simulink model "Bloc_regul_4position_25kHz_discret"  (R2019a)
settings: Solver=VariableStepAuto  StartTime=0.0  StopTime=Tend  RelTol=1e-3
undefined symbols (not defined in the file or in its folder): a1_f, a2_f, b0_f, b1_f, b2_f, d, d_0, d_max, d_min, d_n, Fmax, g, G_f, Jt12, Jt14, Kd_d, Kd_d_sans_int, Kddot_d, Kddot_d_sans_int, Kpi, Kr_d, Kt, Kw_d, Kw_d_sans_int, l, L_n, m, mt, pert, R, tau_ii, tau_md, tau_mi, Udc
libraries: cstblocks x8, simulink x8
settings Model: Creator=Mattia  LastModifiedBy=franc
settings DataIOCC: ReturnWorkspaceOutputs=off
settings DebuggingCC: ArithmeticOperatorsInVariantConditions=warning
settings SFSimCC: SimUseLocalCustomCode=off
settings RTWCC: RTWUseLocalCustomCode=off
settings CodeAppCC: StateflowObjectComments=on

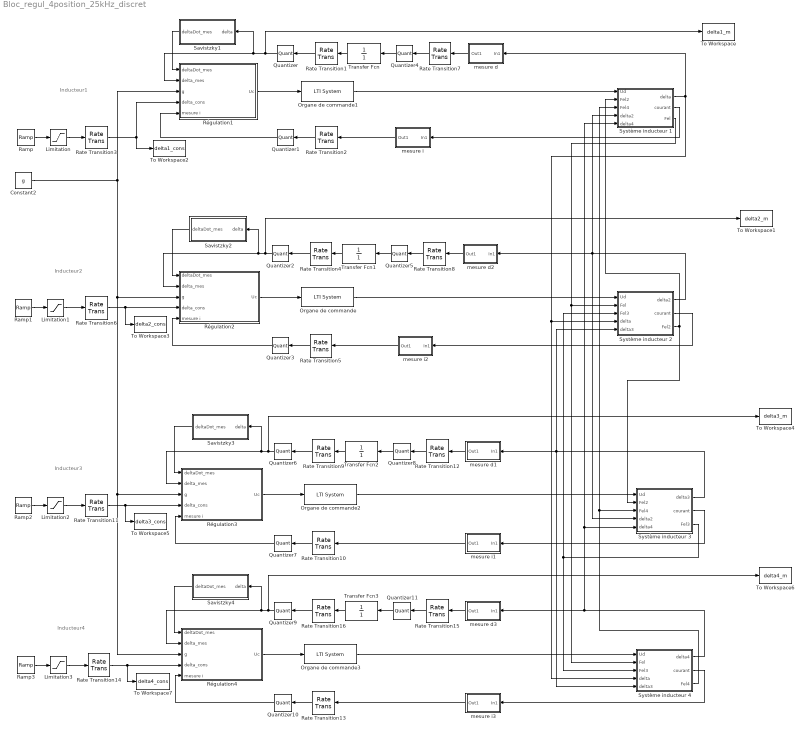
== system Bloc_regul_4position_25kHz_discret ==
  note: Inducteur2
  note: Inducteur1
  note: Inducteur3
  note: Inducteur4
  Constant2 : Constant  Value=g
  Limitation{,1..3} (4 alike) : Saturate  UpperLimit=d_0  LowerLimit=d_n
  Organe de commande{,1..3} (4 alike) : cstblocks/LTI System  sys=Gcm  IC=[]
  Quantizer{,2,6,9} (4 alike) : Quantizer  QuantizationInterval=732e-9
  Quantizer{1,3,7,10} (4 alike) : Quantizer  QuantizationInterval=0.014648438
  Quantizer{4..5,8,11} (4 alike) : Quantizer  QuantizationInterval=6.24e-6
  Ramp : simulink/Sources/Ramp  slope=-0.025  start=0  InitialOutput=d_0
  Ramp1 : simulink/Sources/Ramp  slope=-0.025  start=0.0012  InitialOutput=d_0
  Ramp2 : simulink/Sources/Ramp  slope=-0.025  start=0.4012  InitialOutput=d_0
  Ramp3 : simulink/Sources/Ramp  slope=-0.025  start=0.4  InitialOutput=d_0
  Rate Transition{1..6,9..11,13..14,16} (12 alike) : RateTransition  OutPortSampleTime=h
  Rate Transition{7..8,12,15} (4 alike) : RateTransition  OutPortSampleTime=930e-6
  Régulation1 : Subsystem
  Régulation2 : Subsystem
  Régulation3 : Subsystem
  Régulation4 : Subsystem
  Savistzky1 : Subsystem
  Savistzky2 : Subsystem
  Savistzky3 : Subsystem
  Savistzky4 : Subsystem
  Système inducteur 1 : Subsystem
  Système inducteur 2 : Subsystem
  Système inducteur 3 : Subsystem
  Système inducteur 4 : Subsystem
  To Workspace : ToWorkspace  VariableName=delta1_m  SaveFormat=Timeseries  SampleTime=-1
  To Workspace1 : ToWorkspace  VariableName=delta2_m  SaveFormat=Timeseries  SampleTime=-1
  To Workspace2 : ToWorkspace  VariableName=delta1_cons  SaveFormat=Timeseries  SampleTime=-1
  To Workspace3 : ToWorkspace  VariableName=delta2_cons  SaveFormat=Timeseries  SampleTime=-1
  To Workspace4 : ToWorkspace  VariableName=delta3_m  SaveFormat=Timeseries  SampleTime=-1
  To Workspace5 : ToWorkspace  VariableName=delta3_cons  SaveFormat=Timeseries  SampleTime=-1
  To Workspace6 : ToWorkspace  VariableName=delta4_m  SaveFormat=Timeseries  SampleTime=-1
  To Workspace7 : ToWorkspace  VariableName=delta4_cons  SaveFormat=Timeseries  SampleTime=-1
  Transfer Fcn{,1..3} (4 alike) : TransferFcn  Denominator=[1]
  "mesure d " : Subsystem
  mesure d1 : Subsystem
  mesure d2 : Subsystem
  mesure d3 : Subsystem
  mesure i : Subsystem
  mesure i1 : Subsystem
  mesure i2 : Subsystem
  mesure i3 : Subsystem
  wires:
  Ramp/1 -> Limitation/1
  Limitation/1 -> Rate Transition3/1
  Rate Transition1/1 -> Quantizer/1
  Rate Transition2/1 -> Quantizer1/1
  Limitation1/1 -> Rate Transition6/1
  Rate Transition5/1 -> Quantizer3/1
  Rate Transition4/1 -> Quantizer2/1
  Ramp1/1 -> Limitation1/1
  Quantizer3/1 -> Régulation2/5(mesure i)
  Rate Transition6/1 -> To Workspace3/1, Régulation2/4(delta_cons)
  Constant2/1 -> Régulation3/3(g), Régulation4/3(g), Régulation2/3(g), Régulation1/3(g)
  Rate Transition3/1 -> To Workspace2/1, Régulation1/4(delta_cons)
  Quantizer1/1 -> Régulation1/5(mesure i)
  mesure i/1(Out1) -> Rate Transition2/1
  mesure i2/1(Out1) -> Rate Transition5/1
  Quantizer2/1 -> To Workspace1/1, Régulation2/2(delta_mes), Savistzky2/1(delta)
  Savistzky2/1(deltaDot_mes) -> Régulation2/1(deltaDot_mes)
  Savistzky1/1(deltaDot_mes) -> Régulation1/1(deltaDot_mes)
  Système inducteur 2/2(courant) -> mesure i2/1(In1)
  Système inducteur 1/1(delta) -> Système inducteur 4/4(delta), Système inducteur 2/4(delta), "mesure d "/1(In1)
  Système inducteur 1/2(courant) -> mesure i/1(In1)
  Système inducteur 2/1(delta2) -> Système inducteur 3/4(delta2), Système inducteur 1/4(delta2), mesure d2/1(In1)
  Système inducteur 2/3(Fel2) -> Système inducteur 3/2(Fel2), Système inducteur 1/2(Fel2)
  Organe de commande/1 -> Système inducteur 2/1(Ud)
  Régulation2/1(Uc) -> Organe de commande/1
  Organe de commande1/1 -> Système inducteur 1/1(Ud)
  Régulation1/1(Uc) -> Organe de commande1/1
  Quantizer/1 -> To Workspace/1, Régulation1/2(delta_mes), Savistzky1/1(delta)
  Transfer Fcn/1 -> Rate Transition1/1
  Quantizer4/1 -> Transfer Fcn/1
  Rate Transition7/1 -> Quantizer4/1
  "mesure d "/1(Out1) -> Rate Transition7/1
  mesure d2/1(Out1) -> Rate Transition8/1
  Rate Transition8/1 -> Quantizer5/1
  Quantizer5/1 -> Transfer Fcn1/1
  Transfer Fcn1/1 -> Rate Transition4/1
  Régulation3/1(Uc) -> Organe de commande2/1
  Transfer Fcn2/1 -> Rate Transition9/1
  Rate Transition12/1 -> Quantizer8/1
  Limitation2/1 -> Rate Transition11/1
  Rate Transition10/1 -> Quantizer7/1
  mesure d1/1(Out1) -> Rate Transition12/1
  Quantizer8/1 -> Transfer Fcn2/1
  Organe de commande2/1 -> Système inducteur 3/1(Ud)
  Rate Transition9/1 -> Quantizer6/1
  Système inducteur 3/2(courant) -> mesure i1/1(In1)
  mesure i1/1(Out1) -> Rate Transition10/1
  Quantizer6/1 -> To Workspace4/1, Régulation3/2(delta_mes), Savistzky3/1(delta)
  Ramp2/1 -> Limitation2/1
  Rate Transition11/1 -> To Workspace5/1, Régulation3/4(delta_cons)
  Savistzky3/1(deltaDot_mes) -> Régulation3/1(deltaDot_mes)
  Quantizer7/1 -> Régulation3/5(mesure i)
  Quantizer10/1 -> Régulation4/5(mesure i)
  Rate Transition14/1 -> To Workspace7/1, Régulation4/4(delta_cons)
  Savistzky4/1(deltaDot_mes) -> Régulation4/1(deltaDot_mes)
  Ramp3/1 -> Limitation3/1
  Quantizer9/1 -> To Workspace6/1, Régulation4/2(delta_mes), Savistzky4/1(delta)
  mesure i3/1(Out1) -> Rate Transition13/1
  Système inducteur 4/2(courant) -> mesure i3/1(In1)
  Rate Transition16/1 -> Quantizer9/1
  Rate Transition13/1 -> Quantizer10/1
  Rate Transition15/1 -> Quantizer11/1
  Limitation3/1 -> Rate Transition14/1
  Quantizer11/1 -> Transfer Fcn3/1
  mesure d3/1(Out1) -> Rate Transition15/1
  Transfer Fcn3/1 -> Rate Transition16/1
  Organe de commande3/1 -> Système inducteur 4/1(Ud)
  Régulation4/1(Uc) -> Organe de commande3/1
  Système inducteur 4/3(Fel4) -> Système inducteur 3/3(Fel4), Système inducteur 1/3(Fel4)
  Système inducteur 4/1(delta4) -> Système inducteur 3/5(delta4), Système inducteur 1/5(delta4), mesure d3/1(In1)
  Système inducteur 1/3(Fel) -> Système inducteur 2/2(Fel), Système inducteur 4/2(Fel)
  Système inducteur 3/3(Fel3) -> Système inducteur 2/3(Fel3), Système inducteur 4/3(Fel3)
  Système inducteur 3/1(delta3) -> Système inducteur 4/5(delta3), Système inducteur 2/5(delta3), mesure d1/1(In1)

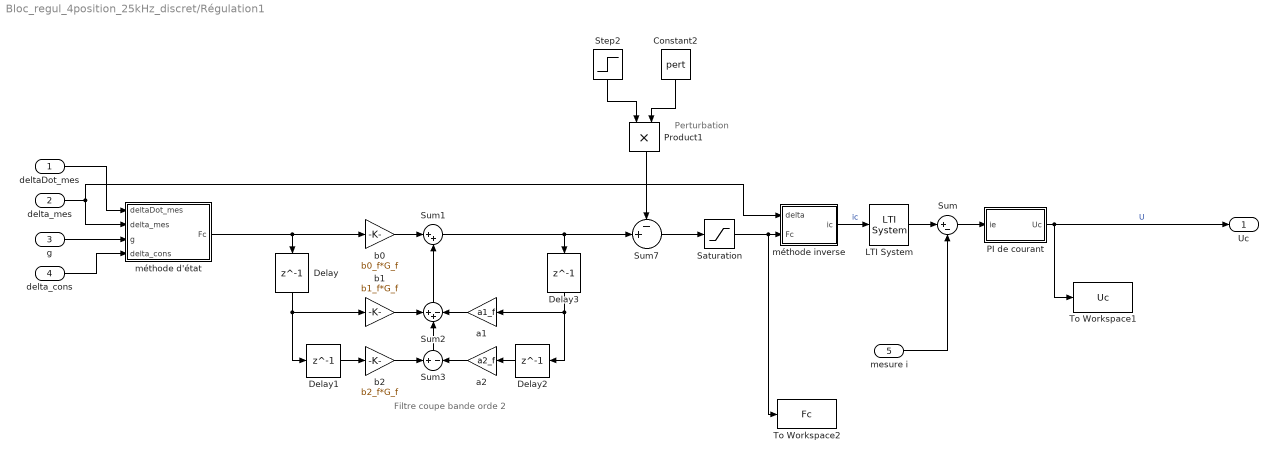
== system Bloc_regul_4position_25kHz_discret/Régulation1 ==
  note: Filtre coupe bande orde 2
  note: Perturbation
  deltaDot_mes : Inport
  delta_mes : Inport  Port=2
  g : Inport  Port=3
  delta_cons : Inport  Port=4
  mesure i : Inport  Port=5
  Constant2 : Constant  Value=pert
  Delay{,1..3} (4 alike) : Delay  DelayLength=1
  LTI System : cstblocks/LTI System  sys=tf(1,1)  IC=[]
  PI de courant : Subsystem
  Product1 : Product
  Saturation : Saturate  UpperLimit=Fmax  LowerLimit=0
  Step2 : Step  After=30  SampleTime=0
  Sum : Sum  Inputs=|+-
  Sum1 : Sum  Inputs=|++
  Sum2 : Sum  Inputs=++-
  Sum3 : Sum  Inputs=+|-
  Sum7 : Sum  Inputs=-+|
  To Workspace1 : ToWorkspace  VariableName=Uc  SaveFormat=Timeseries  SampleTime=-1
  To Workspace2 : ToWorkspace  VariableName=Fc  SaveFormat=Timeseries  SampleTime=-1
  a1 : Gain  Gain=a1_f
  a2 : Gain  Gain=a2_f
  b0 : Gain  Gain=b0_f*G_f
  b1 : Gain  Gain=b1_f*G_f
  b2 : Gain  Gain=b2_f*G_f
  méthode d'état : Subsystem
  méthode inverse : Subsystem
  Uc : Outport
  wires:
  LTI System/1 -> Sum/1
  PI de courant/1(Uc) -> Uc/1, To Workspace1/1  "U"
  Sum/1 -> PI de courant/1(ie)
  méthode inverse/1(ic) -> LTI System/1  "ic"
  mesure i/1 -> Sum/2
  g/1 -> méthode d'état/3("g ")
  delta_cons/1 -> méthode d'état/4(delta_cons)
  delta_mes/1 -> méthode d'état/2(delta_mes), méthode inverse/1(delta)
  deltaDot_mes/1 -> méthode d'état/1(deltaDot_mes)
  méthode d'état/1(Fc) -> b0/1, Delay/1
  b0/1 -> Sum1/1
  a2/1 -> Sum3/2
  Delay3/1 -> a1/1, Delay2/1
  Delay2/1 -> a2/1
  b1/1 -> Sum2/1
  a1/1 -> Sum2/3
  Sum3/1 -> Sum2/2
  Sum2/1 -> Sum1/2
  b2/1 -> Sum3/1
  Delay/1 -> b1/1, Delay1/1
  Delay1/1 -> b2/1
  Saturation/1 -> To Workspace2/1, méthode inverse/2(Fc)
  Sum7/1 -> Saturation/1
  Sum1/1 -> Sum7/2, Delay3/1
  Constant2/1 -> Product1/2
  Step2/1 -> Product1/1
  Product1/1 -> Sum7/1

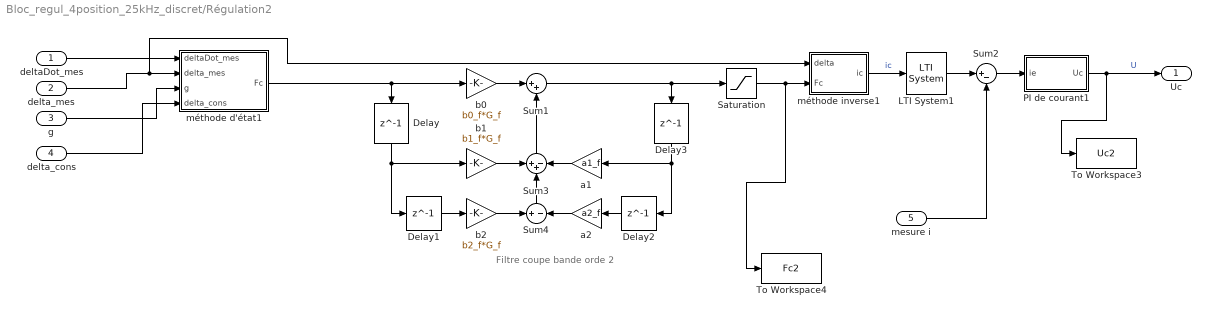
== system Bloc_regul_4position_25kHz_discret/Régulation2 ==
  note: Filtre coupe bande orde 2
  deltaDot_mes : Inport
  delta_mes : Inport  Port=2
  g : Inport  Port=3
  delta_cons : Inport  Port=4
  mesure i : Inport  Port=5
  Delay{,1..3} (4 alike) : Delay  DelayLength=1
  LTI System1 : cstblocks/LTI System  sys=tf(1,1)  IC=[]
  PI de courant1 : Subsystem
  Saturation : Saturate  UpperLimit=Fmax  LowerLimit=0
  Sum1 : Sum  Inputs=|++
  Sum2 : Sum  Inputs=|+-
  Sum3 : Sum  Inputs=++-
  Sum4 : Sum  Inputs=+|-
  To Workspace3 : ToWorkspace  VariableName=Uc2  SaveFormat=Timeseries  SampleTime=-1
  To Workspace4 : ToWorkspace  VariableName=Fc2  SaveFormat=Timeseries  SampleTime=-1
  a1 : Gain  Gain=a1_f
  a2 : Gain  Gain=a2_f
  b0 : Gain  Gain=b0_f*G_f
  b1 : Gain  Gain=b1_f*G_f
  b2 : Gain  Gain=b2_f*G_f
  méthode d'état1 : Subsystem
  méthode inverse1 : Subsystem
  Uc : Outport
  wires:
  PI de courant1/1(Uc) -> Uc/1, To Workspace3/1  "U"
  méthode inverse1/1(ic) -> LTI System1/1  "ic"
  LTI System1/1 -> Sum2/1
  Sum2/1 -> PI de courant1/1(ie)
  deltaDot_mes/1 -> méthode d'état1/1(deltaDot_mes)
  delta_mes/1 -> méthode inverse1/1(delta), méthode d'état1/2(delta_mes)
  g/1 -> méthode d'état1/3("g ")
  delta_cons/1 -> méthode d'état1/4(delta_cons)
  mesure i/1 -> Sum2/2
  b1/1 -> Sum3/1
  Sum3/1 -> Sum1/2
  Delay/1 -> b1/1, Delay1/1
  b2/1 -> Sum4/1
  a2/1 -> Sum4/2
  b0/1 -> Sum1/1
  Delay3/1 -> a1/1, Delay2/1
  Sum4/1 -> Sum3/2
  méthode d'état1/1(Fc) -> b0/1, Delay/1
  a1/1 -> Sum3/3
  Sum1/1 -> Saturation/1, Delay3/1
  Delay2/1 -> a2/1
  Delay1/1 -> b2/1
  Saturation/1 -> To Workspace4/1, méthode inverse1/2(Fc)

== system Bloc_regul_4position_25kHz_discret/Régulation3 ==
  note: Filtre coupe bande orde 2
  deltaDot_mes : Inport
  delta_mes : Inport  Port=2
  g : Inport  Port=3
  delta_cons : Inport  Port=4
  mesure i : Inport  Port=5
  Delay{,1..3} (4 alike) : Delay  DelayLength=1
  LTI System1 : cstblocks/LTI System  sys=tf(1,1)  IC=[]
  PI de courant1 : Subsystem
  Saturation : Saturate  UpperLimit=Fmax  LowerLimit=0
  Sum1 : Sum  Inputs=|++
  Sum2 : Sum  Inputs=|+-
  Sum3 : Sum  Inputs=++-
  Sum4 : Sum  Inputs=+|-
  To Workspace3 : ToWorkspace  VariableName=Uc3  SaveFormat=Timeseries  SampleTime=-1
  To Workspace4 : ToWorkspace  VariableName=Fc3  SaveFormat=Timeseries  SampleTime=-1
  a1 : Gain  Gain=a1_f
  a2 : Gain  Gain=a2_f
  b0 : Gain  Gain=b0_f*G_f
  b1 : Gain  Gain=b1_f*G_f
  b2 : Gain  Gain=b2_f*G_f
  méthode d'état1 : Subsystem
  méthode inverse1 : Subsystem
  Uc : Outport
  wires:
  PI de courant1/1(Uc) -> Uc/1, To Workspace3/1  "U"
  méthode inverse1/1(ic) -> LTI System1/1  "ic"
  LTI System1/1 -> Sum2/1
  Sum2/1 -> PI de courant1/1(ie)
  deltaDot_mes/1 -> méthode d'état1/1(deltaDot_mes)
  delta_mes/1 -> méthode inverse1/1(delta), méthode d'état1/2(delta_mes)
  g/1 -> méthode d'état1/3("g ")
  delta_cons/1 -> méthode d'état1/4(delta_cons)
  mesure i/1 -> Sum2/2
  b1/1 -> Sum3/1
  Sum3/1 -> Sum1/2
  Delay/1 -> b1/1, Delay1/1
  b2/1 -> Sum4/1
  a2/1 -> Sum4/2
  b0/1 -> Sum1/1
  Delay3/1 -> a1/1, Delay2/1
  Sum4/1 -> Sum3/2
  méthode d'état1/1(Fc) -> b0/1, Delay/1
  a1/1 -> Sum3/3
  Sum1/1 -> Saturation/1, Delay3/1
  Delay2/1 -> a2/1
  Delay1/1 -> b2/1
  Saturation/1 -> To Workspace4/1, méthode inverse1/2(Fc)

== system Bloc_regul_4position_25kHz_discret/Régulation4 ==
  note: Filtre coupe bande orde 2
  deltaDot_mes : Inport
  delta_mes : Inport  Port=2
  g : Inport  Port=3
  delta_cons : Inport  Port=4
  mesure i : Inport  Port=5
  Delay{,1..3} (4 alike) : Delay  DelayLength=1
  LTI System1 : cstblocks/LTI System  sys=tf(1,1)  IC=[]
  PI de courant1 : Subsystem
  Saturation : Saturate  UpperLimit=Fmax  LowerLimit=0
  Sum1 : Sum  Inputs=|++
  Sum2 : Sum  Inputs=|+-
  Sum3 : Sum  Inputs=++-
  Sum4 : Sum  Inputs=+|-
  To Workspace3 : ToWorkspace  VariableName=Uc4  SaveFormat=Timeseries  SampleTime=-1
  To Workspace4 : ToWorkspace  VariableName=Fc4  SaveFormat=Timeseries  SampleTime=-1
  a1 : Gain  Gain=a1_f
  a2 : Gain  Gain=a2_f
  b0 : Gain  Gain=b0_f*G_f
  b1 : Gain  Gain=b1_f*G_f
  b2 : Gain  Gain=b2_f*G_f
  méthode d'état1 : Subsystem
  méthode inverse1 : Subsystem
  Uc : Outport
  wires:
  PI de courant1/1(Uc) -> Uc/1, To Workspace3/1  "U"
  méthode inverse1/1(ic) -> LTI System1/1  "ic"
  LTI System1/1 -> Sum2/1
  Sum2/1 -> PI de courant1/1(ie)
  deltaDot_mes/1 -> méthode d'état1/1(deltaDot_mes)
  delta_mes/1 -> méthode inverse1/1(delta), méthode d'état1/2(delta_mes)
  g/1 -> méthode d'état1/3("g ")
  delta_cons/1 -> méthode d'état1/4(delta_cons)
  mesure i/1 -> Sum2/2
  b1/1 -> Sum3/1
  Sum3/1 -> Sum1/2
  Delay/1 -> b1/1, Delay1/1
  b2/1 -> Sum4/1
  a2/1 -> Sum4/2
  b0/1 -> Sum1/1
  Delay3/1 -> a1/1, Delay2/1
  Sum4/1 -> Sum3/2
  méthode d'état1/1(Fc) -> b0/1, Delay/1
  a1/1 -> Sum3/3
  Sum1/1 -> Saturation/1, Delay3/1
  Delay2/1 -> a2/1
  Delay1/1 -> b2/1
  Saturation/1 -> To Workspace4/1, méthode inverse1/2(Fc)

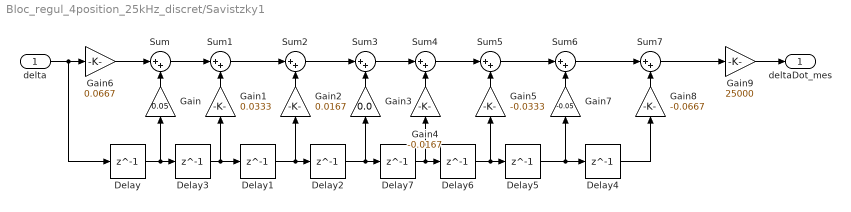
== system Bloc_regul_4position_25kHz_discret/Savistzky1 ==
  delta : Inport
  Delay{,1..7} (8 alike) : Delay  DelayLength=1
  Gain : Gain  Gain=0.05
  Gain1 : Gain  Gain=0.0333
  Gain2 : Gain  Gain=0.0167
  Gain3 : Gain  Gain=0.0
  Gain4 : Gain  Gain=-0.0167
  Gain5 : Gain  Gain=-0.0333
  Gain6 : Gain  Gain=0.0667
  Gain7 : Gain  Gain=-0.05
  Gain8 : Gain  Gain=-0.0667
  Gain9 : Gain  Gain=25000
  Sum{,1..7} (8 alike) : Sum  Inputs=|++
  deltaDot_mes : Outport
  wires:
  Delay6/1 -> Gain5/1, Delay5/1
  Delay2/1 -> Gain3/1, Delay7/1
  Gain9/1 -> deltaDot_mes/1
  Gain/1 -> Sum/2
  Sum/1 -> Sum1/1
  Gain1/1 -> Sum1/2
  Sum1/1 -> Sum2/1
  Gain2/1 -> Sum2/2
  Gain3/1 -> Sum3/2
  Sum3/1 -> Sum4/1
  Gain4/1 -> Sum4/2
  Gain5/1 -> Sum5/2
  Gain7/1 -> Sum6/2
  Gain8/1 -> Sum7/2
  Sum7/1 -> Gain9/1
  Sum6/1 -> Sum7/1
  Sum5/1 -> Sum6/1
  Sum4/1 -> Sum5/1
  Sum2/1 -> Sum3/1
  Delay/1 -> Gain/1, Delay3/1
  Delay3/1 -> Gain1/1, Delay1/1
  Delay4/1 -> Gain8/1
  Delay5/1 -> Gain7/1, Delay4/1
  Delay7/1 -> Gain4/1, Delay6/1
  Delay1/1 -> Gain2/1, Delay2/1
  delta/1 -> Gain6/1, Delay/1
  Gain6/1 -> Sum/1

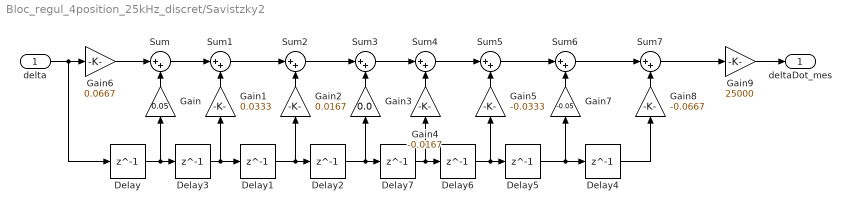
== system Bloc_regul_4position_25kHz_discret/Savistzky2 ==
  delta : Inport
  Delay{,1..7} (8 alike) : Delay  DelayLength=1
  Gain : Gain  Gain=0.05
  Gain1 : Gain  Gain=0.0333
  Gain2 : Gain  Gain=0.0167
  Gain3 : Gain  Gain=0.0
  Gain4 : Gain  Gain=-0.0167
  Gain5 : Gain  Gain=-0.0333
  Gain6 : Gain  Gain=0.0667
  Gain7 : Gain  Gain=-0.05
  Gain8 : Gain  Gain=-0.0667
  Gain9 : Gain  Gain=25000
  Sum{,1..7} (8 alike) : Sum  Inputs=|++
  deltaDot_mes : Outport
  wires:
  Delay6/1 -> Gain5/1, Delay5/1
  Delay2/1 -> Gain3/1, Delay7/1
  Gain9/1 -> deltaDot_mes/1
  Gain/1 -> Sum/2
  Sum/1 -> Sum1/1
  Gain1/1 -> Sum1/2
  Sum1/1 -> Sum2/1
  Gain2/1 -> Sum2/2
  Gain3/1 -> Sum3/2
  Sum3/1 -> Sum4/1
  Gain4/1 -> Sum4/2
  Gain5/1 -> Sum5/2
  Gain7/1 -> Sum6/2
  Gain8/1 -> Sum7/2
  Sum7/1 -> Gain9/1
  Sum6/1 -> Sum7/1
  Sum5/1 -> Sum6/1
  Sum4/1 -> Sum5/1
  Sum2/1 -> Sum3/1
  Delay/1 -> Gain/1, Delay3/1
  Delay3/1 -> Gain1/1, Delay1/1
  Delay4/1 -> Gain8/1
  Delay5/1 -> Gain7/1, Delay4/1
  Delay7/1 -> Gain4/1, Delay6/1
  Delay1/1 -> Gain2/1, Delay2/1
  delta/1 -> Gain6/1, Delay/1
  Gain6/1 -> Sum/1

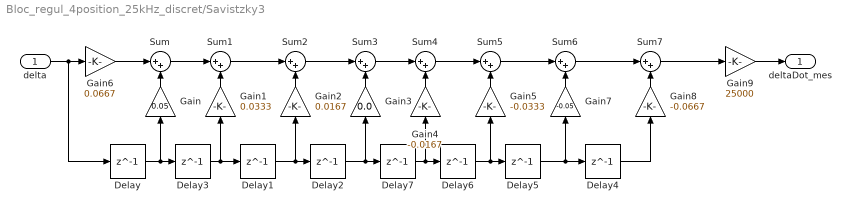
== system Bloc_regul_4position_25kHz_discret/Savistzky3 ==
  delta : Inport
  Delay{,1..7} (8 alike) : Delay  DelayLength=1
  Gain : Gain  Gain=0.05
  Gain1 : Gain  Gain=0.0333
  Gain2 : Gain  Gain=0.0167
  Gain3 : Gain  Gain=0.0
  Gain4 : Gain  Gain=-0.0167
  Gain5 : Gain  Gain=-0.0333
  Gain6 : Gain  Gain=0.0667
  Gain7 : Gain  Gain=-0.05
  Gain8 : Gain  Gain=-0.0667
  Gain9 : Gain  Gain=25000
  Sum{,1..7} (8 alike) : Sum  Inputs=|++
  deltaDot_mes : Outport
  wires:
  Delay6/1 -> Gain5/1, Delay5/1
  Delay2/1 -> Gain3/1, Delay7/1
  Gain9/1 -> deltaDot_mes/1
  Gain/1 -> Sum/2
  Sum/1 -> Sum1/1
  Gain1/1 -> Sum1/2
  Sum1/1 -> Sum2/1
  Gain2/1 -> Sum2/2
  Gain3/1 -> Sum3/2
  Sum3/1 -> Sum4/1
  Gain4/1 -> Sum4/2
  Gain5/1 -> Sum5/2
  Gain7/1 -> Sum6/2
  Gain8/1 -> Sum7/2
  Sum7/1 -> Gain9/1
  Sum6/1 -> Sum7/1
  Sum5/1 -> Sum6/1
  Sum4/1 -> Sum5/1
  Sum2/1 -> Sum3/1
  Delay/1 -> Gain/1, Delay3/1
  Delay3/1 -> Gain1/1, Delay1/1
  Delay4/1 -> Gain8/1
  Delay5/1 -> Gain7/1, Delay4/1
  Delay7/1 -> Gain4/1, Delay6/1
  Delay1/1 -> Gain2/1, Delay2/1
  delta/1 -> Gain6/1, Delay/1
  Gain6/1 -> Sum/1

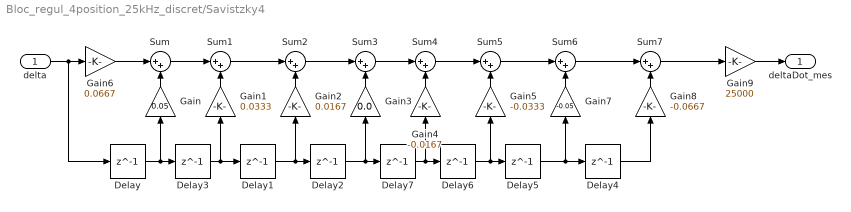
== system Bloc_regul_4position_25kHz_discret/Savistzky4 ==
  delta : Inport
  Delay{,1..7} (8 alike) : Delay  DelayLength=1
  Gain : Gain  Gain=0.05
  Gain1 : Gain  Gain=0.0333
  Gain2 : Gain  Gain=0.0167
  Gain3 : Gain  Gain=0.0
  Gain4 : Gain  Gain=-0.0167
  Gain5 : Gain  Gain=-0.0333
  Gain6 : Gain  Gain=0.0667
  Gain7 : Gain  Gain=-0.05
  Gain8 : Gain  Gain=-0.0667
  Gain9 : Gain  Gain=25000
  Sum{,1..7} (8 alike) : Sum  Inputs=|++
  deltaDot_mes : Outport
  wires:
  Delay6/1 -> Gain5/1, Delay5/1
  Delay2/1 -> Gain3/1, Delay7/1
  Gain9/1 -> deltaDot_mes/1
  Gain/1 -> Sum/2
  Sum/1 -> Sum1/1
  Gain1/1 -> Sum1/2
  Sum1/1 -> Sum2/1
  Gain2/1 -> Sum2/2
  Gain3/1 -> Sum3/2
  Sum3/1 -> Sum4/1
  Gain4/1 -> Sum4/2
  Gain5/1 -> Sum5/2
  Gain7/1 -> Sum6/2
  Gain8/1 -> Sum7/2
  Sum7/1 -> Gain9/1
  Sum6/1 -> Sum7/1
  Sum5/1 -> Sum6/1
  Sum4/1 -> Sum5/1
  Sum2/1 -> Sum3/1
  Delay/1 -> Gain/1, Delay3/1
  Delay3/1 -> Gain1/1, Delay1/1
  Delay4/1 -> Gain8/1
  Delay5/1 -> Gain7/1, Delay4/1
  Delay7/1 -> Gain4/1, Delay6/1
  Delay1/1 -> Gain2/1, Delay2/1
  delta/1 -> Gain6/1, Delay/1
  Gain6/1 -> Sum/1

== system Bloc_regul_4position_25kHz_discret/Système inducteur 1 ==
  Ud : Inport
  Fel2 : Inport  Port=2
  Fel4 : Inport  Port=3
  delta2 : Inport  Port=4
  delta4 : Inport  Port=5
  Partie Electrique : Subsystem
  Partie Mécanique : Subsystem
  delta : Outport
  courant : Outport  Port=2
  Fel : Outport  Port=3
  wires:
  Ud/1 -> Partie Electrique/1(Ud)
  Partie Mécanique/2(delta) -> Partie Electrique/3(delta), delta/1
  Partie Electrique/1(i) -> courant/1
  Partie Mécanique/1(deltaDot) -> Partie Electrique/2(deltaDot)
  Partie Electrique/2(Fel) -> Fel/1, Partie Mécanique/1(Fel)
  Fel2/1 -> Partie Mécanique/2(Fel2)
  delta2/1 -> Partie Mécanique/4(delta2)
  Fel4/1 -> Partie Mécanique/3(Fel4)
  delta4/1 -> Partie Mécanique/5(delta4)

== system Bloc_regul_4position_25kHz_discret/Système inducteur 2 ==
  Ud : Inport
  Fel : Inport  Port=2
  Fel3 : Inport  Port=3
  delta : Inport  Port=4
  delta3 : Inport  Port=5
  Partie Electrique : Subsystem
  Partie Mécanique2 : Subsystem
  delta2 : Outport
  courant : Outport  Port=2
  Fel2 : Outport  Port=3
  wires:
  Ud/1 -> Partie Electrique/1(Ud)
  Partie Mécanique2/2(delta2) -> Partie Electrique/3(delta), delta2/1
  Partie Electrique/1(i2) -> courant/1
  Partie Mécanique2/1(deltaDot2) -> Partie Electrique/2(deltaDot)
  Partie Electrique/2(Fel2) -> Fel2/1, Partie Mécanique2/2(Fel2)
  Fel/1 -> Partie Mécanique2/1(Fel)
  delta/1 -> Partie Mécanique2/4(Delta)
  Fel3/1 -> Partie Mécanique2/3(Fel3)
  delta3/1 -> Partie Mécanique2/5(Delta3)

== system Bloc_regul_4position_25kHz_discret/Système inducteur 3 ==
  Ud : Inport
  Fel2 : Inport  Port=2
  Fel4 : Inport  Port=3
  delta2 : Inport  Port=4
  delta4 : Inport  Port=5
  Partie Electrique : Subsystem
  Partie Mécanique2 : Subsystem
  delta3 : Outport
  courant : Outport  Port=2
  Fel3 : Outport  Port=3
  wires:
  Ud/1 -> Partie Electrique/1(Ud)
  Partie Mécanique2/2(delta3) -> Partie Electrique/3(delta), delta3/1
  Partie Electrique/1(i3) -> courant/1
  Partie Mécanique2/1(deltaDot3) -> Partie Electrique/2(deltaDot)
  Partie Electrique/2(Fel3) -> Fel3/1, Partie Mécanique2/2(Fel3)
  Fel2/1 -> Partie Mécanique2/1(Fel2)
  delta2/1 -> Partie Mécanique2/4(Delta2)
  Fel4/1 -> Partie Mécanique2/3(Fel4)
  delta4/1 -> Partie Mécanique2/5(Delta4)

== system Bloc_regul_4position_25kHz_discret/Système inducteur 4 ==
  Ud : Inport
  Fel : Inport  Port=2
  Fel3 : Inport  Port=3
  delta : Inport  Port=4
  delta3 : Inport  Port=5
  Partie Electrique : Subsystem
  Partie Mécanique2 : Subsystem
  delta4 : Outport
  courant : Outport  Port=2
  Fel4 : Outport  Port=3
  wires:
  Ud/1 -> Partie Electrique/1(Ud)
  Partie Mécanique2/2(delta4) -> Partie Electrique/3(delta), delta4/1
  Partie Electrique/1(i4) -> courant/1
  Partie Mécanique2/1(deltaDot4) -> Partie Electrique/2(deltaDot)
  Partie Electrique/2(Fel4) -> Partie Mécanique2/3(Fel4), Fel4/1
  Fel/1 -> Partie Mécanique2/1(Fel)
  delta/1 -> Partie Mécanique2/4(Delta)
  Fel3/1 -> Partie Mécanique2/2(Fel3)
  delta3/1 -> Partie Mécanique2/5(Delta3)

== system Bloc_regul_4position_25kHz_discret/mesure d  ==
  In1 : Inport
  Gain : Gain  Gain=1/tau_md
  Integrator : Integrator  InitialCondition=d_0
  Sum : Sum  Inputs=|+-
  Out1 : Outport
  wires:
  Gain/1 -> Integrator/1
  Integrator/1 -> Sum/2, Out1/1
  In1/1 -> Sum/1
  Sum/1 -> Gain/1

== system Bloc_regul_4position_25kHz_discret/mesure d1 ==
  In1 : Inport
  Gain : Gain  Gain=1/tau_md
  Integrator : Integrator  InitialCondition=d_0
  Sum : Sum  Inputs=|+-
  Out1 : Outport
  wires:
  Gain/1 -> Integrator/1
  Integrator/1 -> Sum/2, Out1/1
  In1/1 -> Sum/1
  Sum/1 -> Gain/1

== system Bloc_regul_4position_25kHz_discret/mesure d2 ==
  In1 : Inport
  Gain : Gain  Gain=1/tau_md
  Integrator : Integrator  InitialCondition=d_0
  Sum : Sum  Inputs=|+-
  Out1 : Outport
  wires:
  Gain/1 -> Integrator/1
  Integrator/1 -> Sum/2, Out1/1
  In1/1 -> Sum/1
  Sum/1 -> Gain/1

== system Bloc_regul_4position_25kHz_discret/mesure d3 ==
  In1 : Inport
  Gain : Gain  Gain=1/tau_md
  Integrator : Integrator  InitialCondition=d_0
  Sum : Sum  Inputs=|+-
  Out1 : Outport
  wires:
  Gain/1 -> Integrator/1
  Integrator/1 -> Sum/2, Out1/1
  In1/1 -> Sum/1
  Sum/1 -> Gain/1

== system Bloc_regul_4position_25kHz_discret/mesure i ==
  In1 : Inport
  Gain : Gain  Gain=1/tau_mi
  Integrator : Integrator
  Sum : Sum  Inputs=|+-
  Out1 : Outport
  wires:
  Gain/1 -> Integrator/1
  In1/1 -> Sum/1
  Integrator/1 -> Sum/2, Out1/1
  Sum/1 -> Gain/1

== system Bloc_regul_4position_25kHz_discret/mesure i1 ==
  In1 : Inport
  Gain : Gain  Gain=1/tau_mi
  Integrator : Integrator
  Sum : Sum  Inputs=|+-
  Out1 : Outport
  wires:
  Gain/1 -> Integrator/1
  In1/1 -> Sum/1
  Integrator/1 -> Sum/2, Out1/1
  Sum/1 -> Gain/1

== system Bloc_regul_4position_25kHz_discret/mesure i2 ==
  In1 : Inport
  Gain : Gain  Gain=1/tau_mi
  Integrator : Integrator
  Sum : Sum  Inputs=|+-
  Out1 : Outport
  wires:
  Gain/1 -> Integrator/1
  In1/1 -> Sum/1
  Integrator/1 -> Sum/2, Out1/1
  Sum/1 -> Gain/1

== system Bloc_regul_4position_25kHz_discret/mesure i3 ==
  In1 : Inport
  Gain : Gain  Gain=1/tau_mi
  Integrator : Integrator
  Sum : Sum  Inputs=|+-
  Out1 : Outport
  wires:
  Gain/1 -> Integrator/1
  In1/1 -> Sum/1
  Integrator/1 -> Sum/2, Out1/1
  Sum/1 -> Gain/1

== system Bloc_regul_4position_25kHz_discret/Régulation1/PI de courant ==
  ie : Inport
  Gain : Gain  Gain=Kpi
  Gain1 : Gain  Gain=1/tau_ii
  Integrator : Integrator
  Saturation : Saturate  UpperLimit=Udc  LowerLimit=0
  Sum : Sum  Inputs=|++
  Sum1 : Sum  Inputs=|+-
  Sum4 : Sum  Inputs=+|-
  Uc : Outport
  wires:
  Sum1/1 -> Gain1/1
  Saturation/1 -> Sum4/2, Uc/1
  Sum/1 -> Saturation/1, Sum4/1
  Integrator/1 -> Sum/2
  Gain/1 -> Sum1/1, Sum/1
  Gain1/1 -> Integrator/1
  Sum4/1 -> Sum1/2
  ie/1 -> Gain/1

== system Bloc_regul_4position_25kHz_discret/Régulation1/méthode d'état ==
  deltaDot_mes : Inport
  delta_mes : Inport  Port=2
  "g " : Inport  Port=3
  delta_cons : Inport  Port=4
  Delay : Delay  DelayLength=1  InitialCondition=0
  Gain : Gain  Gain=m
  Gain1 : Gain  Gain=Kw_d
  Gain2 : Gain  Gain=Kr_d
  Gain3 : Gain  Gain=Kddot_d
  Gain4 : Gain  Gain=Kd_d
  Gain5 : Gain  Gain=1/Kw_d
  Saturation : Saturate  UpperLimit=Fmax  LowerLimit=0
  Sum : Sum  Inputs=+++
  Sum1 : Sum  Inputs=+-
  Sum2 : Sum  Inputs=|++
  Sum3 : Sum  Inputs=+-|
  Sum4 : Sum  Inputs=+|-
  Sum5 : Sum  Inputs=|+-
  Sum6 : Sum  Inputs=|++
  To Workspace1 : ToWorkspace  VariableName=Reg_cons  SaveFormat=Timeseries  SampleTime=-1
  To Workspace2 : ToWorkspace  VariableName=MG  SaveFormat=Timeseries  SampleTime=-1
  To Workspace3 : ToWorkspace  VariableName=Integrateur  SaveFormat=Timeseries  SampleTime=-1
  To Workspace4 : ToWorkspace  VariableName=Fc_reg  SaveFormat=Timeseries  SampleTime=-1
  Fc : Outport
  wires:
  Sum5/1 -> Sum6/1
  deltaDot_mes/1 -> Gain3/1
  delta_mes/1 -> Gain4/1, Sum1/2
  delta_cons/1 -> Sum1/1, Gain1/1
  Delay/1 -> Sum6/2, Gain2/1
  "g "/1 -> Gain/1
  Saturation/1 -> Fc/1, Sum4/2
  Sum6/1 -> Delay/1
  Gain4/1 -> Sum2/1
  Gain2/1 -> Sum3/1
  Gain/1 -> Sum/1, To Workspace2/1
  Gain3/1 -> Sum2/2
  Gain5/1 -> Sum5/2
  Sum2/1 -> Sum3/2
  Sum4/1 -> Gain5/1
  Sum3/1 -> To Workspace3/1, Sum/3
  Sum1/1 -> Sum5/1
  Gain1/1 -> To Workspace1/1, Sum/2
  Sum/1 -> To Workspace4/1, Sum4/1, Saturation/1

== system Bloc_regul_4position_25kHz_discret/Régulation1/méthode inverse ==
  delta : Inport
  Fc : Inport  Port=2
  Gain : Gain  Gain=2/(L_n*d_n)
  Product : Product
  Sqrt : Sqrt  OutputSignalType=real  SaturateOnIntegerOverflow=on
  ic : Outport
  wires:
  Gain/1 -> Sqrt/1
  Fc/1 -> Gain/1
  delta/1 -> Product/1
  Product/1 -> ic/1
  Sqrt/1 -> Product/2

== system Bloc_regul_4position_25kHz_discret/Régulation2/PI de courant1 ==
  ie : Inport
  Gain : Gain  Gain=Kpi
  Gain1 : Gain  Gain=1/tau_ii
  Integrator : Integrator
  Saturation : Saturate  UpperLimit=Udc  LowerLimit=0
  Sum : Sum  Inputs=|++
  Sum1 : Sum  Inputs=|+-
  Sum4 : Sum  Inputs=+|-
  Uc : Outport
  wires:
  Sum1/1 -> Gain1/1
  Saturation/1 -> Sum4/2, Uc/1
  Sum/1 -> Saturation/1, Sum4/1
  Integrator/1 -> Sum/2
  Gain/1 -> Sum1/1, Sum/1
  Gain1/1 -> Integrator/1
  Sum4/1 -> Sum1/2
  ie/1 -> Gain/1

== system Bloc_regul_4position_25kHz_discret/Régulation2/méthode d'état1 ==
  deltaDot_mes : Inport
  delta_mes : Inport  Port=2
  "g " : Inport  Port=3
  delta_cons : Inport  Port=4
  Delay : Delay  DelayLength=1  InitialCondition=0
  Gain : Gain  Gain=m
  Gain1 : Gain  Gain=Kw_d
  Gain2 : Gain  Gain=Kr_d
  Gain3 : Gain  Gain=Kddot_d
  Gain4 : Gain  Gain=Kd_d
  Gain5 : Gain  Gain=1/Kw_d
  Saturation : Saturate  UpperLimit=Fmax  LowerLimit=0
  Sum : Sum  Inputs=+++
  Sum1 : Sum  Inputs=+-
  Sum2 : Sum  Inputs=|++
  Sum3 : Sum  Inputs=+-|
  Sum4 : Sum  Inputs=+|-
  Sum5 : Sum  Inputs=|+-
  Sum6 : Sum  Inputs=|++
  Fc : Outport
  wires:
  Sum5/1 -> Sum6/1
  deltaDot_mes/1 -> Gain3/1
  delta_mes/1 -> Gain4/1, Sum1/2
  delta_cons/1 -> Sum1/1, Gain1/1
  Delay/1 -> Sum6/2, Gain2/1
  "g "/1 -> Gain/1
  Saturation/1 -> Fc/1, Sum4/2
  Sum6/1 -> Delay/1
  Gain4/1 -> Sum2/1
  Gain2/1 -> Sum3/1
  Gain/1 -> Sum/1
  Gain3/1 -> Sum2/2
  Gain5/1 -> Sum5/2
  Sum2/1 -> Sum3/2
  Sum4/1 -> Gain5/1
  Sum3/1 -> Sum/3
  Sum1/1 -> Sum5/1
  Gain1/1 -> Sum/2
  Sum/1 -> Sum4/1, Saturation/1

== system Bloc_regul_4position_25kHz_discret/Régulation2/méthode inverse1 ==
  delta : Inport
  Fc : Inport  Port=2
  Gain : Gain  Gain=2/(L_n*d_n)
  Product : Product
  Sqrt : Sqrt  OutputSignalType=real  SaturateOnIntegerOverflow=on
  ic : Outport
  wires:
  Gain/1 -> Sqrt/1
  Fc/1 -> Gain/1
  delta/1 -> Product/1
  Product/1 -> ic/1
  Sqrt/1 -> Product/2

== system Bloc_regul_4position_25kHz_discret/Régulation3/PI de courant1 ==
  ie : Inport
  Gain : Gain  Gain=Kpi
  Gain1 : Gain  Gain=1/tau_ii
  Integrator : Integrator
  Saturation : Saturate  UpperLimit=Udc  LowerLimit=0
  Sum : Sum  Inputs=|++
  Sum1 : Sum  Inputs=|+-
  Sum4 : Sum  Inputs=+|-
  Uc : Outport
  wires:
  Sum1/1 -> Gain1/1
  Saturation/1 -> Sum4/2, Uc/1
  Sum/1 -> Saturation/1, Sum4/1
  Integrator/1 -> Sum/2
  Gain/1 -> Sum1/1, Sum/1
  Gain1/1 -> Integrator/1
  Sum4/1 -> Sum1/2
  ie/1 -> Gain/1

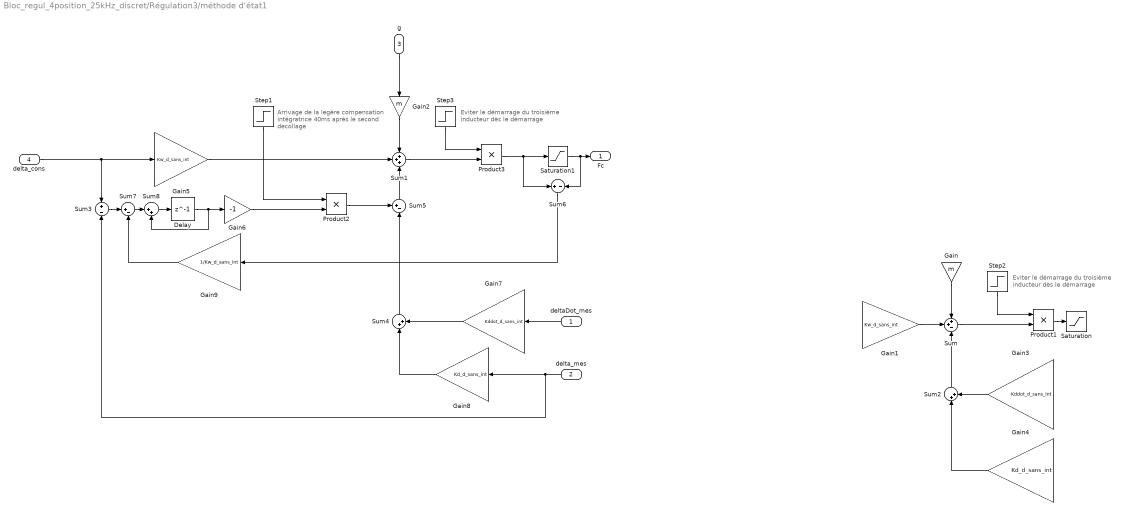
== system Bloc_regul_4position_25kHz_discret/Régulation3/méthode d'état1 ==
  note: Eviter le démarrage du troisième
      | inducteur dès le démarrage
  note: Eviter le démarrage du troisième
      | inducteur dès le démarrage
  note: Arrivage de la legère compensation
      | intégratrice 40ms après le second
      | decollage
  deltaDot_mes : Inport
  delta_mes : Inport  Port=2
  "g " : Inport  Port=3
  delta_cons : Inport  Port=4
  Delay : Delay  DelayLength=1  InitialCondition=0
  Gain : Gain  Gain=m
  Gain1 : Gain  Gain=Kw_d_sans_int
  Gain2 : Gain  Gain=m
  Gain3 : Gain  Gain=Kddot_d_sans_int
  Gain4 : Gain  Gain=Kd_d_sans_int
  Gain5 : Gain  Gain=Kw_d_sans_int
  Gain6 : Gain  Gain=-1
  Gain7 : Gain  Gain=Kddot_d_sans_int
  Gain8 : Gain  Gain=Kd_d_sans_int
  Gain9 : Gain  Gain=1/Kw_d_sans_int
  Product1 : Product
  Product2 : Product
  Product3 : Product
  Saturation : Saturate  UpperLimit=Fmax  LowerLimit=0
  Saturation1 : Saturate  UpperLimit=Fmax  LowerLimit=0
  Step1 : Step  Time=0.440  SampleTime=0
  Step2 : Step  Time=0.4  SampleTime=0
  Step3 : Step  Time=0.4  SampleTime=0
  Sum : Sum  Inputs=++-
  Sum1 : Sum  Inputs=+++
  Sum2 : Sum  Inputs=|++
  Sum3 : Sum  Inputs=+-
  Sum4 : Sum  Inputs=|++
  Sum5 : Sum  Inputs=+-|
  Sum6 : Sum  Inputs=+|-
  Sum7 : Sum  Inputs=|+-
  Sum8 : Sum  Inputs=|++
  Fc : Outport
  wires:
  "g "/1 -> Gain2/1
  deltaDot_mes/1 -> Gain7/1
  Sum8/1 -> Delay/1
  delta_mes/1 -> Sum3/2, Gain8/1
  delta_cons/1 -> Gain5/1, Sum3/1
  Sum4/1 -> Sum5/2
  Sum5/1 -> Sum1/3
  Sum7/1 -> Sum8/1
  Delay/1 -> Sum8/2, Gain6/1
  Gain2/1 -> Sum1/1
  Gain9/1 -> Sum7/2
  Gain8/1 -> Sum4/1
  Gain5/1 -> Sum1/2
  Sum3/1 -> Sum7/1
  Sum6/1 -> Gain9/1
  Gain7/1 -> Sum4/2
  Sum1/1 -> Product3/2
  Step3/1 -> Product3/1
  Product3/1 -> Sum6/1, Saturation1/1
  Product1/1 -> Saturation/1
  ? -> Gain1/1
  ? -> Gain3/1
  Gain3/1 -> Sum2/2
  Sum/1 -> Product1/2
  Sum2/1 -> Sum/3
  ? -> Gain4/1
  Gain1/1 -> Sum/2
  Gain4/1 -> Sum2/1
  Step2/1 -> Product1/1
  Gain/1 -> Sum/1
  ? -> Gain/1
  Saturation1/1 -> Sum6/2, Fc/1
  Step1/1 -> Product2/1
  Gain6/1 -> Product2/2
  Product2/1 -> Sum5/1

== system Bloc_regul_4position_25kHz_discret/Régulation3/méthode inverse1 ==
  delta : Inport
  Fc : Inport  Port=2
  Gain : Gain  Gain=2/(L_n*d_n)
  Product : Product
  Sqrt : Sqrt  OutputSignalType=real  SaturateOnIntegerOverflow=on
  ic : Outport
  wires:
  Gain/1 -> Sqrt/1
  Fc/1 -> Gain/1
  delta/1 -> Product/1
  Product/1 -> ic/1
  Sqrt/1 -> Product/2

== system Bloc_regul_4position_25kHz_discret/Régulation4/PI de courant1 ==
  ie : Inport
  Gain : Gain  Gain=Kpi
  Gain1 : Gain  Gain=1/tau_ii
  Integrator : Integrator
  Saturation : Saturate  UpperLimit=Udc  LowerLimit=0
  Sum : Sum  Inputs=|++
  Sum1 : Sum  Inputs=|+-
  Sum4 : Sum  Inputs=+|-
  Uc : Outport
  wires:
  Sum1/1 -> Gain1/1
  Saturation/1 -> Sum4/2, Uc/1
  Sum/1 -> Saturation/1, Sum4/1
  Integrator/1 -> Sum/2
  Gain/1 -> Sum1/1, Sum/1
  Gain1/1 -> Integrator/1
  Sum4/1 -> Sum1/2
  ie/1 -> Gain/1

== system Bloc_regul_4position_25kHz_discret/Régulation4/méthode d'état1 ==
  deltaDot_mes : Inport
  delta_mes : Inport  Port=2
  "g " : Inport  Port=3
  delta_cons : Inport  Port=4
  Delay : Delay  DelayLength=1  InitialCondition=0
  Gain : Gain  Gain=m
  Gain1 : Gain  Gain=Kw_d
  Gain2 : Gain  Gain=Kr_d
  Gain3 : Gain  Gain=Kddot_d
  Gain4 : Gain  Gain=Kd_d
  Gain5 : Gain  Gain=1/Kw_d
  Saturation : Saturate  UpperLimit=Fmax  LowerLimit=0
  Sum : Sum  Inputs=+++
  Sum1 : Sum  Inputs=+-
  Sum2 : Sum  Inputs=|++
  Sum3 : Sum  Inputs=+-|
  Sum4 : Sum  Inputs=+|-
  Sum5 : Sum  Inputs=|+-
  Sum6 : Sum  Inputs=|++
  Fc : Outport
  wires:
  Sum5/1 -> Sum6/1
  deltaDot_mes/1 -> Gain3/1
  delta_mes/1 -> Gain4/1, Sum1/2
  delta_cons/1 -> Sum1/1, Gain1/1
  Delay/1 -> Sum6/2, Gain2/1
  "g "/1 -> Gain/1
  Saturation/1 -> Fc/1, Sum4/2
  Sum6/1 -> Delay/1
  Gain4/1 -> Sum2/1
  Gain2/1 -> Sum3/1
  Gain/1 -> Sum/1
  Gain3/1 -> Sum2/2
  Gain5/1 -> Sum5/2
  Sum2/1 -> Sum3/2
  Sum4/1 -> Gain5/1
  Sum3/1 -> Sum/3
  Sum1/1 -> Sum5/1
  Gain1/1 -> Sum/2
  Sum/1 -> Sum4/1, Saturation/1

== system Bloc_regul_4position_25kHz_discret/Régulation4/méthode inverse1 ==
  delta : Inport
  Fc : Inport  Port=2
  Gain : Gain  Gain=2/(L_n*d_n)
  Product : Product
  Sqrt : Sqrt  OutputSignalType=real  SaturateOnIntegerOverflow=on
  ic : Outport
  wires:
  Gain/1 -> Sqrt/1
  Fc/1 -> Gain/1
  delta/1 -> Product/1
  Product/1 -> ic/1
  Sqrt/1 -> Product/2

== system Bloc_regul_4position_25kHz_discret/Système inducteur 1/Partie Electrique ==
  Ud : Inport
  deltaDot : Inport  Port=2
  delta : Inport  Port=3
  Divide : Product  Inputs=*/  CollapseMode=Specified dimension
  Gain : Gain  Gain=R
  Gain1 : Gain  Gain=1/(L_n*d_n)
  Gain3 : Gain  Gain=L_n*d_n/2
  Integrator : Integrator
  Product : Product
  Product1 : Product
  Square : Math  Operator=square  RndMeth=Zero  SaturateOnIntegerOverflow=on
  Sum : Sum  Inputs=-+|
  Sum1 : Sum  Inputs=|++
  To Workspace1 : ToWorkspace  VariableName=Fel  SaveFormat=Timeseries  SampleTime=-1
  To Workspace3 : ToWorkspace  VariableName=i  SaveFormat=Timeseries  SampleTime=-1
  i : Outport
  Fel : Outport  Port=2
  wires:
  deltaDot/1 -> Product1/2  "deltaDot"
  Gain/1 -> Sum/1
  Ud/1 -> Sum/2  "Ud"
  Divide/1 -> Square/1, Product1/1
  Product1/1 -> Sum1/2
  Gain1/1 -> Product/1
  Integrator/1 -> To Workspace3/1, i/1, Divide/1, Gain/1  "i"
  Sum1/1 -> Integrator/1  "di/dt"
  Product/1 -> Sum1/1
  Sum/1 -> Gain1/1
  Square/1 -> Gain3/1
  delta/1 -> Product/2, Divide/2  "delta"
  Gain3/1 -> To Workspace1/1, Fel/1  "Fel"

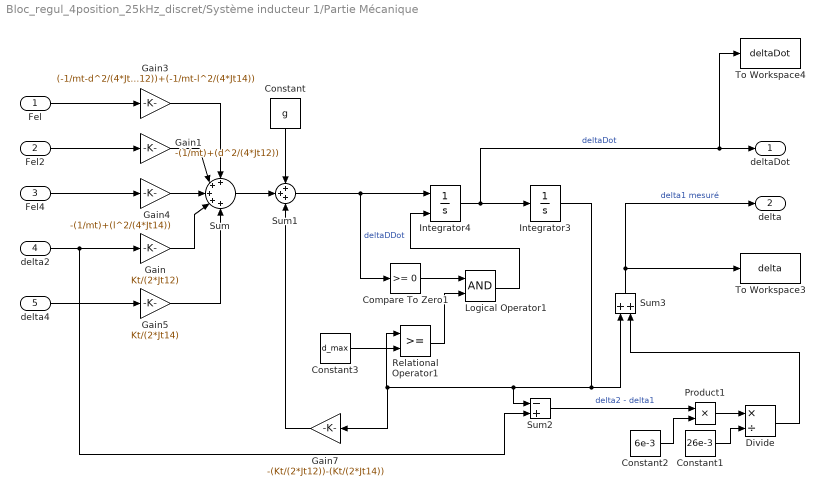
== system Bloc_regul_4position_25kHz_discret/Système inducteur 1/Partie Mécanique ==
  Fel : Inport
  Fel2 : Inport  Port=2
  Fel4 : Inport  Port=3
  delta2 : Inport  Port=4
  delta4 : Inport  Port=5
  Compare To Zero1 : simulink/Logic and Bit Operations/Compare To Zero  relop=>=  OutDataTypeStr=boolean
  Constant : Constant  Value=g
  Constant1 : Constant  Value=26e-3
  Constant2 : Constant  Value=6e-3
  Constant3 : Constant  Value=d_max
  Divide : Product  Inputs=*/
  Gain : Gain  Gain=Kt/(2*Jt12)
  Gain1 : Gain  Gain=-(1/mt)+(d^2/(4*Jt12))
  Gain3 : Gain  Gain=(-1/mt-d^2/(4*Jt12))+(-1/mt-l^2/(4*Jt14))
  Gain4 : Gain  Gain=-(1/mt)+(l^2/(4*Jt14))
  Gain5 : Gain  Gain=Kt/(2*Jt14)
  Gain7 : Gain  Gain=-(Kt/(2*Jt12))-(Kt/(2*Jt14))
  Integrator3 : Integrator  InitialCondition=d_0  LimitOutput=on  UpperSaturationLimit=d_max  LowerSaturationLimit=d_min
  Integrator4 : Integrator  ExternalReset=level  UpperSaturationLimit=0
  Logical Operator1 : Logic  AllPortsSameDT=off  OutDataTypeStr=boolean
  Product1 : Product
  Relational Operator1 : RelationalOperator  OutDataTypeStr=boolean  RndMeth=Simplest
  Sum : Sum  Inputs=+++++
  Sum1 : Sum  Inputs=+++
  Sum2 : Sum  Inputs=-+
  Sum3 : Sum
  To Workspace3 : ToWorkspace  VariableName=delta  SaveFormat=Timeseries  SampleTime=-1
  To Workspace4 : ToWorkspace  VariableName=deltaDot  SaveFormat=Timeseries  SampleTime=-1
  deltaDot : Outport
  delta : Outport  Port=2
  wires:
  Sum1/1 -> Compare To Zero1/1, Integrator4/1  "deltaDDot"
  Integrator4/1 -> To Workspace4/1, deltaDot/1, Integrator3/1  "deltaDot"
  Integrator3/1 -> Sum3/1, Sum2/1, Gain7/1, Relational Operator1/1
  Constant3/1 -> Relational Operator1/2
  Compare To Zero1/1 -> Logical Operator1/1
  Logical Operator1/1 -> Integrator4/2
  Relational Operator1/1 -> Logical Operator1/2
  Gain7/1 -> Sum1/3
  Constant/1 -> Sum1/1
  Sum/1 -> Sum1/2
  Gain1/1 -> Sum/2
  Fel2/1 -> Gain1/1
  delta2/1 -> Sum2/2, Gain/1
  Gain/1 -> Sum/4
  delta4/1 -> Gain5/1
  Fel/1 -> Gain3/1
  Gain3/1 -> Sum/1
  Fel4/1 -> Gain4/1
  Gain4/1 -> Sum/3
  Gain5/1 -> Sum/5
  Divide/1 -> Sum3/2
  Sum2/1 -> Product1/1  "delta2 - delta1"
  Product1/1 -> Divide/1
  Constant1/1 -> Divide/2
  Constant2/1 -> Product1/2
  Sum3/1 -> To Workspace3/1, delta/1  "delta1 mesuré"

== system Bloc_regul_4position_25kHz_discret/Système inducteur 2/Partie Electrique ==
  Ud : Inport
  deltaDot : Inport  Port=2
  delta : Inport  Port=3
  Divide : Product  Inputs=*/  CollapseMode=Specified dimension
  Gain : Gain  Gain=R
  Gain1 : Gain  Gain=1/(L_n*d_n)
  Gain3 : Gain  Gain=L_n*d_n/2
  Integrator : Integrator
  Product : Product
  Product1 : Product
  Square : Math  Operator=square  RndMeth=Zero  SaturateOnIntegerOverflow=on
  Sum : Sum  Inputs=-+|
  Sum1 : Sum  Inputs=|++
  To Workspace1 : ToWorkspace  VariableName=Fel2  SaveFormat=Timeseries  SampleTime=-1
  To Workspace3 : ToWorkspace  VariableName=i2  SaveFormat=Timeseries  SampleTime=-1
  i2 : Outport
  Fel2 : Outport  Port=2
  wires:
  deltaDot/1 -> Product1/2  "deltaDot"
  Gain/1 -> Sum/1
  Ud/1 -> Sum/2  "Ud"
  Divide/1 -> Square/1, Product1/1
  Product1/1 -> Sum1/2
  Gain1/1 -> Product/1
  Integrator/1 -> To Workspace3/1, i2/1, Divide/1, Gain/1  "i"
  Sum1/1 -> Integrator/1  "di/dt"
  Product/1 -> Sum1/1
  Sum/1 -> Gain1/1
  Square/1 -> Gain3/1
  delta/1 -> Product/2, Divide/2  "delta"
  Gain3/1 -> To Workspace1/1, Fel2/1  "Fel"

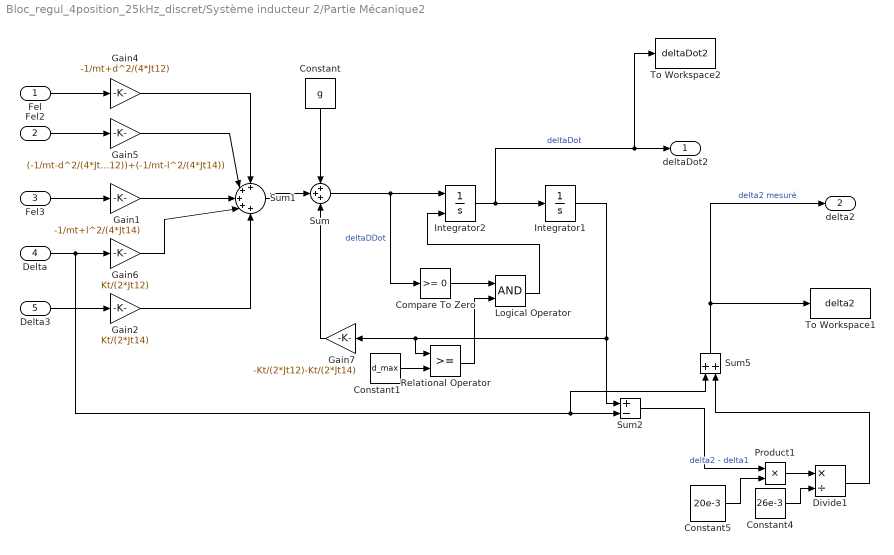
== system Bloc_regul_4position_25kHz_discret/Système inducteur 2/Partie Mécanique2 ==
  Fel : Inport
  Fel2 : Inport  Port=2
  Fel3 : Inport  Port=3
  Delta : Inport  Port=4
  Delta3 : Inport  Port=5
  Compare To Zero : simulink/Logic and Bit Operations/Compare To Zero  relop=>=  OutDataTypeStr=boolean
  Constant : Constant  Value=g
  Constant1 : Constant  Value=d_max
  Constant4 : Constant  Value=26e-3
  Constant5 : Constant  Value=20e-3
  Divide1 : Product  Inputs=*/
  Gain1 : Gain  Gain=-1/mt+l^2/(4*Jt14)
  Gain2 : Gain  Gain=Kt/(2*Jt14)
  Gain4 : Gain  Gain=-1/mt+d^2/(4*Jt12)
  Gain5 : Gain  Gain=(-1/mt-d^2/(4*Jt12))+(-1/mt-l^2/(4*Jt14))
  Gain6 : Gain  Gain=Kt/(2*Jt12)
  Gain7 : Gain  Gain=-Kt/(2*Jt12)-Kt/(2*Jt14)
  Integrator1 : Integrator  InitialCondition=d_0  LimitOutput=on  UpperSaturationLimit=d_max  LowerSaturationLimit=d_min
  Integrator2 : Integrator  ExternalReset=level  UpperSaturationLimit=0
  Logical Operator : Logic  AllPortsSameDT=off  OutDataTypeStr=boolean
  Product1 : Product
  Relational Operator : RelationalOperator  OutDataTypeStr=boolean  RndMeth=Simplest
  Sum : Sum  Inputs=+++
  Sum1 : Sum  Inputs=+++++
  Sum2 : Sum  Inputs=+-
  Sum5 : Sum
  To Workspace1 : ToWorkspace  VariableName=delta2  SaveFormat=Timeseries  SampleTime=-1
  To Workspace2 : ToWorkspace  VariableName=deltaDot2  SaveFormat=Timeseries  SampleTime=-1
  deltaDot2 : Outport
  delta2 : Outport  Port=2
  wires:
  Sum/1 -> Compare To Zero/1, Integrator2/1  "deltaDDot"
  Relational Operator/1 -> Logical Operator/2
  Integrator2/1 -> To Workspace2/1, deltaDot2/1, Integrator1/1  "deltaDot"
  Integrator1/1 -> Sum2/1, Relational Operator/1, Gain7/1
  Compare To Zero/1 -> Logical Operator/1
  Logical Operator/1 -> Integrator2/2
  Constant1/1 -> Relational Operator/2
  Gain5/1 -> Sum1/2
  Gain4/1 -> Sum1/1
  Delta/1 -> Sum2/2, Sum5/1, Gain6/1
  Fel2/1 -> Gain5/1
  Fel/1 -> Gain4/1
  Sum1/1 -> Sum/2
  Gain7/1 -> Sum/3
  Constant/1 -> Sum/1
  Fel3/1 -> Gain1/1
  Gain6/1 -> Sum1/4
  Delta3/1 -> Gain2/1
  Gain1/1 -> Sum1/3
  Gain2/1 -> Sum1/5
  Sum2/1 -> Product1/1  "delta2 - delta1"
  Constant4/1 -> Divide1/2
  Constant5/1 -> Product1/2
  Divide1/1 -> Sum5/2
  Product1/1 -> Divide1/1
  Sum5/1 -> To Workspace1/1, delta2/1  "delta2 mesuré"

== system Bloc_regul_4position_25kHz_discret/Système inducteur 3/Partie Electrique ==
  Ud : Inport
  deltaDot : Inport  Port=2
  delta : Inport  Port=3
  Divide : Product  Inputs=*/  CollapseMode=Specified dimension
  Gain : Gain  Gain=R
  Gain1 : Gain  Gain=1/(L_n*d_n)
  Gain3 : Gain  Gain=L_n*d_n/2
  Integrator : Integrator
  Product : Product
  Product1 : Product
  Square : Math  Operator=square  RndMeth=Zero  SaturateOnIntegerOverflow=on
  Sum : Sum  Inputs=-+|
  Sum1 : Sum  Inputs=|++
  To Workspace1 : ToWorkspace  VariableName=Fel3  SaveFormat=Timeseries  SampleTime=-1
  To Workspace3 : ToWorkspace  VariableName=i3  SaveFormat=Timeseries  SampleTime=-1
  i3 : Outport
  Fel3 : Outport  Port=2
  wires:
  deltaDot/1 -> Product1/2  "deltaDot"
  Gain/1 -> Sum/1
  Ud/1 -> Sum/2  "Ud"
  Divide/1 -> Square/1, Product1/1
  Product1/1 -> Sum1/2
  Gain1/1 -> Product/1
  Integrator/1 -> To Workspace3/1, i3/1, Divide/1, Gain/1  "i"
  Sum1/1 -> Integrator/1  "di/dt"
  Product/1 -> Sum1/1
  Sum/1 -> Gain1/1
  Square/1 -> Gain3/1
  delta/1 -> Product/2, Divide/2  "delta"
  Gain3/1 -> To Workspace1/1, Fel3/1  "Fel"

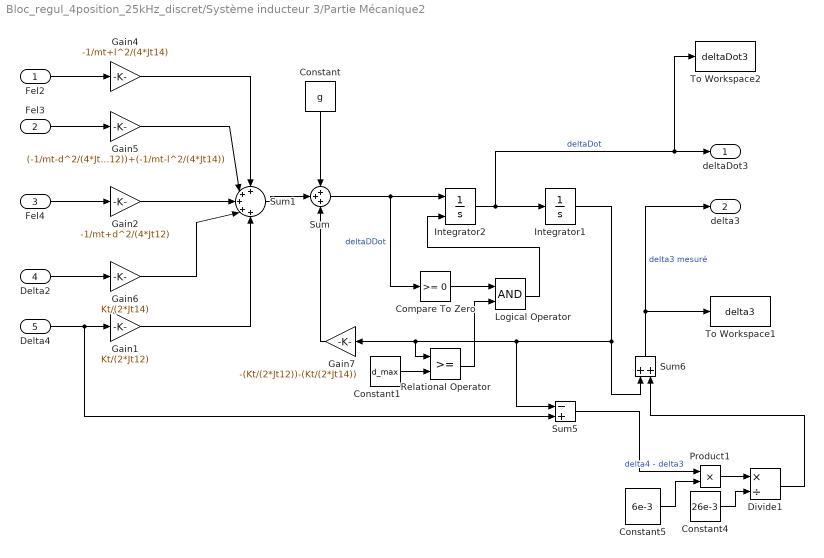
== system Bloc_regul_4position_25kHz_discret/Système inducteur 3/Partie Mécanique2 ==
  Fel2 : Inport
  Fel3 : Inport  Port=2
  Fel4 : Inport  Port=3
  Delta2 : Inport  Port=4
  Delta4 : Inport  Port=5
  Compare To Zero : simulink/Logic and Bit Operations/Compare To Zero  relop=>=  OutDataTypeStr=boolean
  Constant : Constant  Value=g
  Constant1 : Constant  Value=d_max
  Constant4 : Constant  Value=26e-3
  Constant5 : Constant  Value=6e-3
  Divide1 : Product  Inputs=*/
  Gain1 : Gain  Gain=Kt/(2*Jt12)
  Gain2 : Gain  Gain=-1/mt+d^2/(4*Jt12)
  Gain4 : Gain  Gain=-1/mt+l^2/(4*Jt14)
  Gain5 : Gain  Gain=(-1/mt-d^2/(4*Jt12))+(-1/mt-l^2/(4*Jt14))
  Gain6 : Gain  Gain=Kt/(2*Jt14)
  Gain7 : Gain  Gain=-(Kt/(2*Jt12))-(Kt/(2*Jt14))
  Integrator1 : Integrator  InitialCondition=d_0  LimitOutput=on  UpperSaturationLimit=d_max  LowerSaturationLimit=d_min
  Integrator2 : Integrator  ExternalReset=level  UpperSaturationLimit=0
  Logical Operator : Logic  AllPortsSameDT=off  OutDataTypeStr=boolean
  Product1 : Product
  Relational Operator : RelationalOperator  OutDataTypeStr=boolean  RndMeth=Simplest
  Sum : Sum  Inputs=+++
  Sum1 : Sum  Inputs=+++++
  Sum5 : Sum  Inputs=-+
  Sum6 : Sum
  To Workspace1 : ToWorkspace  VariableName=delta3  SaveFormat=Timeseries  SampleTime=-1
  To Workspace2 : ToWorkspace  VariableName=deltaDot3  SaveFormat=Timeseries  SampleTime=-1
  deltaDot3 : Outport
  delta3 : Outport  Port=2
  wires:
  Sum/1 -> Compare To Zero/1, Integrator2/1  "deltaDDot"
  Relational Operator/1 -> Logical Operator/2
  Integrator2/1 -> To Workspace2/1, deltaDot3/1, Integrator1/1  "deltaDot"
  Integrator1/1 -> Sum6/1, Sum5/1, Relational Operator/1, Gain7/1
  Compare To Zero/1 -> Logical Operator/1
  Logical Operator/1 -> Integrator2/2
  Constant1/1 -> Relational Operator/2
  Gain5/1 -> Sum1/2
  Delta2/1 -> Gain6/1
  Fel3/1 -> Gain5/1
  Fel2/1 -> Gain4/1
  Sum1/1 -> Sum/2
  Gain7/1 -> Sum/3
  Constant/1 -> Sum/1
  Delta4/1 -> Sum5/2, Gain1/1
  Fel4/1 -> Gain2/1
  Gain2/1 -> Sum1/3
  Gain1/1 -> Sum1/5
  Gain4/1 -> Sum1/1
  Gain6/1 -> Sum1/4
  Constant5/1 -> Product1/2
  Sum5/1 -> Product1/1  "delta4 - delta3"
  Divide1/1 -> Sum6/2
  Product1/1 -> Divide1/1
  Constant4/1 -> Divide1/2
  Sum6/1 -> To Workspace1/1, delta3/1  "delta3 mesuré"

== system Bloc_regul_4position_25kHz_discret/Système inducteur 4/Partie Electrique ==
  Ud : Inport
  deltaDot : Inport  Port=2
  delta : Inport  Port=3
  Divide : Product  Inputs=*/  CollapseMode=Specified dimension
  Gain : Gain  Gain=R
  Gain1 : Gain  Gain=1/(L_n*d_n)
  Gain3 : Gain  Gain=L_n*d_n/2
  Integrator : Integrator
  Product : Product
  Product1 : Product
  Square : Math  Operator=square  RndMeth=Zero  SaturateOnIntegerOverflow=on
  Sum : Sum  Inputs=-+|
  Sum1 : Sum  Inputs=|++
  To Workspace1 : ToWorkspace  VariableName=Fel4  SaveFormat=Timeseries  SampleTime=-1
  To Workspace3 : ToWorkspace  VariableName=i4  SaveFormat=Timeseries  SampleTime=-1
  i4 : Outport
  Fel4 : Outport  Port=2
  wires:
  deltaDot/1 -> Product1/2  "deltaDot"
  Gain/1 -> Sum/1
  Ud/1 -> Sum/2  "Ud"
  Divide/1 -> Square/1, Product1/1
  Product1/1 -> Sum1/2
  Gain1/1 -> Product/1
  Integrator/1 -> To Workspace3/1, i4/1, Divide/1, Gain/1  "i"
  Sum1/1 -> Integrator/1  "di/dt"
  Product/1 -> Sum1/1
  Sum/1 -> Gain1/1
  Square/1 -> Gain3/1
  delta/1 -> Product/2, Divide/2  "delta"
  Gain3/1 -> To Workspace1/1, Fel4/1  "Fel"

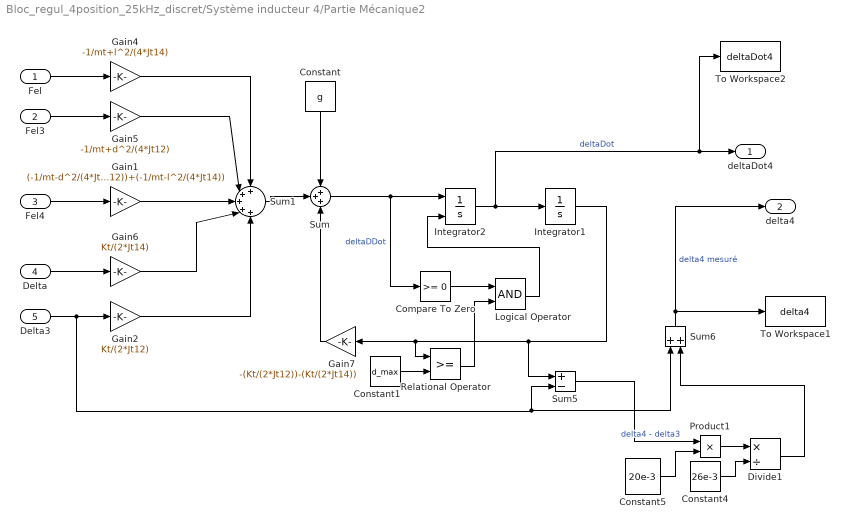
== system Bloc_regul_4position_25kHz_discret/Système inducteur 4/Partie Mécanique2 ==
  Fel : Inport
  Fel3 : Inport  Port=2
  Fel4 : Inport  Port=3
  Delta : Inport  Port=4
  Delta3 : Inport  Port=5
  Compare To Zero : simulink/Logic and Bit Operations/Compare To Zero  relop=>=  OutDataTypeStr=boolean
  Constant : Constant  Value=g
  Constant1 : Constant  Value=d_max
  Constant4 : Constant  Value=26e-3
  Constant5 : Constant  Value=20e-3
  Divide1 : Product  Inputs=*/
  Gain1 : Gain  Gain=(-1/mt-d^2/(4*Jt12))+(-1/mt-l^2/(4*Jt14))
  Gain2 : Gain  Gain=Kt/(2*Jt12)
  Gain4 : Gain  Gain=-1/mt+l^2/(4*Jt14)
  Gain5 : Gain  Gain=-1/mt+d^2/(4*Jt12)
  Gain6 : Gain  Gain=Kt/(2*Jt14)
  Gain7 : Gain  Gain=-(Kt/(2*Jt12))-(Kt/(2*Jt14))
  Integrator1 : Integrator  InitialCondition=d_0  LimitOutput=on  UpperSaturationLimit=d_max  LowerSaturationLimit=d_min
  Integrator2 : Integrator  ExternalReset=level  UpperSaturationLimit=0
  Logical Operator : Logic  AllPortsSameDT=off  OutDataTypeStr=boolean
  Product1 : Product
  Relational Operator : RelationalOperator  OutDataTypeStr=boolean  RndMeth=Simplest
  Sum : Sum  Inputs=+++
  Sum1 : Sum  Inputs=+++++
  Sum5 : Sum  Inputs=+-
  Sum6 : Sum
  To Workspace1 : ToWorkspace  VariableName=delta4  SaveFormat=Timeseries  SampleTime=-1
  To Workspace2 : ToWorkspace  VariableName=deltaDot4  SaveFormat=Timeseries  SampleTime=-1
  deltaDot4 : Outport
  delta4 : Outport  Port=2
  wires:
  Sum/1 -> Compare To Zero/1, Integrator2/1  "deltaDDot"
  Relational Operator/1 -> Logical Operator/2
  Integrator2/1 -> To Workspace2/1, deltaDot4/1, Integrator1/1  "deltaDot"
  Integrator1/1 -> Sum5/1, Relational Operator/1, Gain7/1
  Compare To Zero/1 -> Logical Operator/1
  Logical Operator/1 -> Integrator2/2
  Constant1/1 -> Relational Operator/2
  Gain5/1 -> Sum1/2
  Delta/1 -> Gain6/1
  Fel3/1 -> Gain5/1
  Fel/1 -> Gain4/1
  Sum1/1 -> Sum/2
  Gain7/1 -> Sum/3
  Constant/1 -> Sum/1
  Fel4/1 -> Gain1/1
  Gain1/1 -> Sum1/3
  Delta3/1 -> Sum6/1, Sum5/2, Gain2/1
  Gain2/1 -> Sum1/5
  Gain4/1 -> Sum1/1
  Gain6/1 -> Sum1/4
  Constant5/1 -> Product1/2
  Sum5/1 -> Product1/1  "delta4 - delta3"
  Divide1/1 -> Sum6/2
  Product1/1 -> Divide1/1
  Constant4/1 -> Divide1/2
  Sum6/1 -> delta4/1, To Workspace1/1  "delta4 mesuré"
